simulink model "w1prob5"  (R2020a)
settings: Solver=VariableStepAuto  StartTime=0.0  StopTime=10.0  RelTol=1e-3
undefined symbols (not defined in the file): ic
libraries: simulink x1
settings Model: Creator=Anjali123  LastModifiedBy=Anjali123

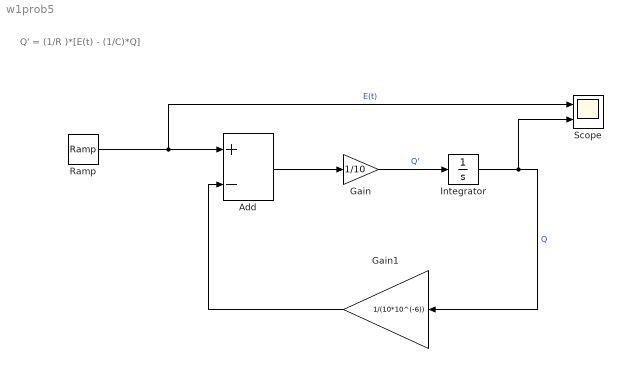
== system w1prob5 ==
  note: Q' = (1/R )*[E(t) - (1/C)*Q]
  Add : Sum  Inputs=+-
  Gain : Gain  Gain=1/10
  Gain1 : Gain  Gain=1/(10*10^(-6))
  Integrator : Integrator  InitialCondition=ic
  Ramp : simulink/Sources/Ramp  slope=1  start=0  InitialOutput=0
  Scope : Scope  NumInputPorts=2
  wires:
  Ramp/1 -> Scope/1, Add/1  "E(t)"
  Add/1 -> Gain/1
  Gain/1 -> Integrator/1  "Q'"
  Integrator/1 -> Scope/2, Gain1/1  "Q"
  Gain1/1 -> Add/2
